simulink model "Rocket_Launch_Sim"  (R2023b)
settings: Solver=VariableStepAuto  StartTime=0.0  StopTime=30  RelTol=1e-3
values from neighbouring files (symbols this model uses):
  A = 10.75    [RocketParameters.m]
  Cd = 0.3    [RocketParameters.m]
  pitch_0 = 0    [RocketParameters.m]
  rho = 1.225    [RocketParameters.m]
  roll_0 = 0    [RocketParameters.m]
  Thrust = 7607000    [RocketParameters.m]
  yaw_0 = 0    [RocketParameters.m]
settings Model: Creator=Mia Morrison  LastModifiedBy=Mia Morrison

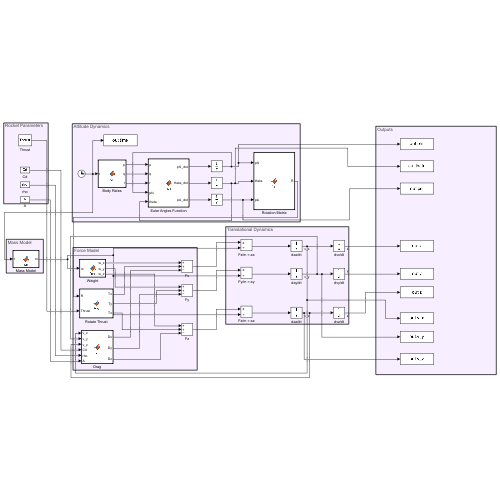
[thumbnail: Simulink's stored preview of the top-level diagram]
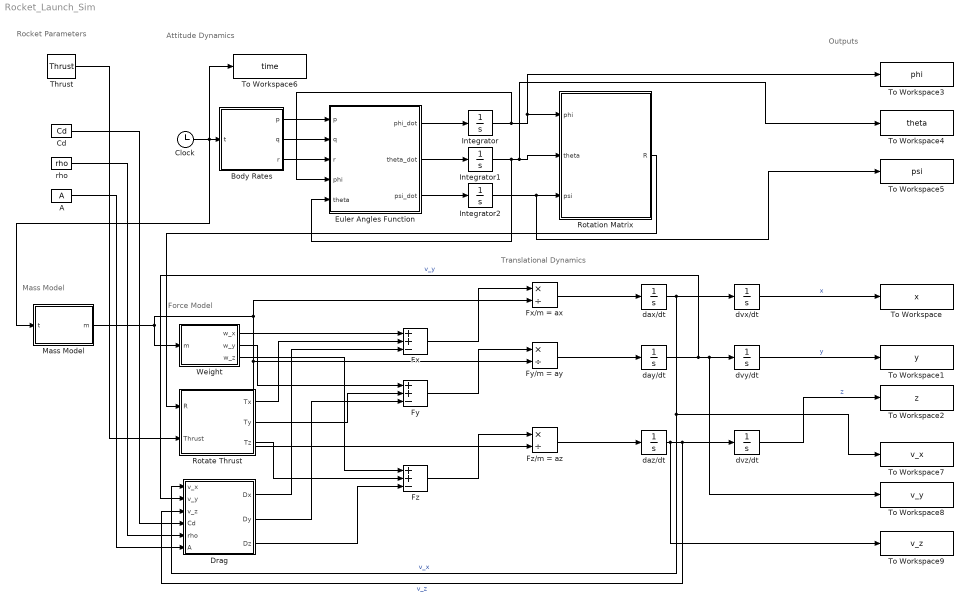
== system Rocket_Launch_Sim ==
  note: Outputs
  note: Translational Dynamics
  note: Force Model
  note: Rocket Parameters
  note: Mass Model
  note: Attitude Dynamics
  A : Constant  Value=A
  Body Rates : MATLAB Function  TreatAsAtomicUnit=on
  Cd : Constant  Value=Cd
  Clock : Clock
  Drag : MATLAB Function  TreatAsAtomicUnit=on
  Euler Angles Function : MATLAB Function  TreatAsAtomicUnit=on
  Fx : Sum  Inputs=++-
  Fx/m = ax : Product  Inputs=*/
  Fy : Sum  Inputs=++-
  Fy/m = ay : Product  Inputs=*/
  Fz : Sum  Inputs=++-
  Fz/m = az : Product  Inputs=*/
  Integrator : Integrator  InitialCondition=roll_0
  Integrator1 : Integrator  InitialCondition=pitch_0
  Integrator2 : Integrator  InitialCondition=yaw_0
  Mass Model : MATLAB Function  TreatAsAtomicUnit=on
  Rotate Thrust : MATLAB Function  TreatAsAtomicUnit=on
  Rotation Matrix : MATLAB Function  TreatAsAtomicUnit=on
  Thrust : Constant  Value=Thrust
  To Workspace : ToWorkspace  VariableName=x  SampleTime=-1
  To Workspace1 : ToWorkspace  VariableName=y  SampleTime=-1
  To Workspace2 : ToWorkspace  VariableName=z  SampleTime=-1
  To Workspace3 : ToWorkspace  VariableName=phi  SampleTime=-1
  To Workspace4 : ToWorkspace  VariableName=theta  SampleTime=-1
  To Workspace5 : ToWorkspace  VariableName=psi  SampleTime=-1
  To Workspace6 : ToWorkspace  VariableName=time  SampleTime=-1
  To Workspace7 : ToWorkspace  VariableName=v_x  SampleTime=-1
  To Workspace8 : ToWorkspace  VariableName=v_y  SampleTime=-1
  To Workspace9 : ToWorkspace  VariableName=v_z  SampleTime=-1
  Weight : MATLAB Function  TreatAsAtomicUnit=on
  dax/dt : Integrator
  day/dt : Integrator
  daz/dt : Integrator
  dvx/dt : Integrator
  dvy/dt : Integrator
  dvz/dt : Integrator
  rho : Constant  Value=rho
  wires:
  Euler Angles Function/3(psi_dot) -> Integrator2/1
  Euler Angles Function/1(phi_dot) -> Integrator/1
  Euler Angles Function/2(theta_dot) -> Integrator1/1
  Body Rates/2(q) -> Euler Angles Function/2(q)
  Body Rates/1(p) -> Euler Angles Function/1(p)
  Body Rates/3(r) -> Euler Angles Function/3(r)
  Clock/1 -> Mass Model/1(t), Body Rates/1(t), To Workspace6/1
  rho/1 -> Drag/5(rho)
  Cd/1 -> Drag/4(Cd)
  A/1 -> Drag/6(A)
  Rotation Matrix/1(R) -> Rotate Thrust/1(R)
  Drag/2(Dy) -> Fy/3
  Rotate Thrust/1(Tx) -> Fx/2
  Weight/1(w_x) -> Fx/1
  Drag/1(Dx) -> Fx/3
  Thrust/1 -> Rotate Thrust/2(Thrust)
  Rotate Thrust/3(Tz) -> Fz/2
  Weight/2(w_y) -> Fy/1
  Rotate Thrust/2(Ty) -> Fy/2
  Weight/3(w_z) -> Fz/1
  Drag/3(Dz) -> Fz/3
  Fy/1 -> Fy/m = ay/1
  Fx/1 -> Fx/m = ax/1
  Fz/1 -> Fz/m = az/1
  daz/dt/1 -> dvz/dt/1, Drag/3(v_z), To Workspace9/1  "v_z"
  dvy/dt/1 -> To Workspace1/1  "y"
  dax/dt/1 -> To Workspace7/1, Drag/1(v_x), dvx/dt/1  "v_x"
  day/dt/1 -> dvy/dt/1, To Workspace8/1, Drag/2(v_y)  "v_y"
  dvz/dt/1 -> To Workspace2/1  "z"
  Fx/m = ax/1 -> dax/dt/1
  dvx/dt/1 -> To Workspace/1  "x"
  Fy/m = ay/1 -> day/dt/1
  Mass Model/1(m) -> Weight/1(m), Fz/m = az/2, Fy/m = ay/2, Fx/m = ax/2
  Fz/m = az/1 -> daz/dt/1
  Integrator2/1 -> To Workspace5/1, Rotation Matrix/3(psi)
  Integrator/1 -> To Workspace3/1, Rotation Matrix/1(phi), Euler Angles Function/4(phi)
  Integrator1/1 -> To Workspace4/1, Rotation Matrix/2(theta), Euler Angles Function/5(theta)

== matlab function Rocket_Launch_Sim/Rotation Matrix ==
  data: phi input; R output; theta input; psi input
function R  = fcn(phi,theta,psi)

% Rotation matrix. Given EA, which direction is the rocket pointing?

% 3-2-1 rotation

cphi = cos(phi);
sphi = sin(phi);

cth = cos(theta);
sth = sin(theta);

cpsi = cos(psi);
spsi = sin(psi);

R_z = [cpsi, -spsi, 0; spsi, cpsi, 0; 0, 0, 1];
R_y = [cth, 0, sth; 0, 1, 0; -sth, 0, cth];
R_x = [1, 0, 0; 0, cphi, -sphi; 0, sphi, cphi];


R = R_z * R_y * R_x;

== matlab function Rocket_Launch_Sim/Mass Model ==
  data: t input; m output
function m = fcn(t)

m_0 = 549054;      % kg
m_dry = 25600;     % kg
burn_time = 162;    % sec

m_dot = (m_0 - m_dry)/burn_time; 

if t < burn_time
    m = m_0 - m_dot*t;
else 
    m = m_dry;
end

== matlab function Rocket_Launch_Sim/Drag ==
  data: v_x input; v_y input; v_z input; Dx output; Cd input; rho input; A input; Dy output; Dz output
function [Dx,Dy,Dz] = fcn(v_x,v_y,v_z,Cd,rho,A)

% Drag

V = sqrt(v_x^2 + v_y^2 + v_z^2);

if V < 1e-6
    Dx = 0;
    Dy = 0;
    Dz = 0;
else
    D = 0.5*rho*Cd*A*V^2;

    Dx = -D*v_x/V;
    Dy = -D*v_y/V;
    Dz = -D*v_z/V;
end

end

== matlab function Rocket_Launch_Sim/Euler Angles Function ==
  data: p input; phi_dot output; theta_dot output; psi_dot output; q input; r input; phi input; theta input
function [phi_dot, theta_dot, psi_dot] = fcn(p, q, r, phi, theta)

% Euler Angles

% p = roll rate. q = pitch rate. r = yaw rate

phi_dot = p + q*sin(phi)*tan(theta) + r*cos(phi)*tan(theta);

theta_dot = q*cos(phi) - r*sin(phi);

psi_dot = q*sin(phi)/cos(theta) + r*cos(phi)/cos(theta);

end

== matlab function Rocket_Launch_Sim/Body Rates ==
  data: t input; p output; q output; r output
function [p, q, r] = fcn(t)

p = 0;
r = 0;

if t < 5
    q = 0;
elseif t < 15
    q = -0.02;   % rad/s (pitch over)
else
    q = 0;
end

end

== matlab function Rocket_Launch_Sim/Rotate Thrust ==
  data: R input; Tx output; Thrust input; Ty output; Tz output
function [Tx, Ty, Tz] = fcn(R, Thrust)

T_body = [0; 0; Thrust];

T_world = R*T_body;

Tx = T_world(1);
Ty = T_world(2);
Tz = T_world(3);

end

== matlab function Rocket_Launch_Sim/Weight ==
  data: m input; w_x output; w_y output; w_z output
function [w_x, w_y, w_z] = fcn(m)

w_x = 0;
w_y = 0;
w_z = -m * 9.81 ;

end
